simulink model "rozniczka"  (Simulink 7.1)
settings: Solver=ode45  StartTime=0.0  StopTime=10.0  MaxStep=0.1  MinStep=0.001  RelTol=1e-3
settings Model: Creator=surbaniak  LastModifiedBy=surbaniak

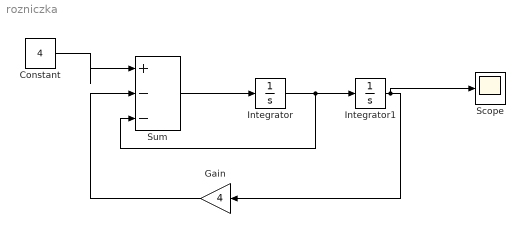
== system rozniczka ==
  Constant : Constant  Value=4  OutDataType=sfix(16)  OutScaling=2^0
  Gain : Gain  Orientation=left  Gain=4  ParameterDataType=sfix(16)  ParameterScaling=2^0  OutDataType=sfix(16)  OutScaling=2^0
  Integrator : Integrator
  Integrator1 : Integrator
  Scope : Scope
  Sum : Sum  Inputs=|+--  OutDataType=sfix(16)  OutScaling=2^0
  wires:
  Constant/1 -> Sum/1
  Sum/1 -> Integrator/1
  Integrator/1 -> Integrator1/1, Sum/3
  Integrator1/1 -> Gain/1, Scope/1
  Gain/1 -> Sum/2
